simulink model "Vector_ComplexMult_Ex1"  (R2024a)
settings: Solver=VariableStepAuto  StartTime=0.0  StopTime=10  RelTol=1e-3
undefined symbols (not defined in the file): i, L, vsva2197, xcvc1702
libraries: hdlSSR x5, hdlBasic x4, vmcUtilities x1
settings Model: Creator=robg  LastModifiedBy=sdegala

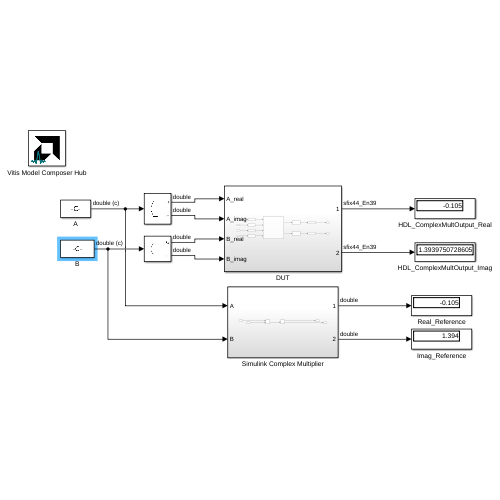
[thumbnail: Simulink's stored preview of the top-level diagram]
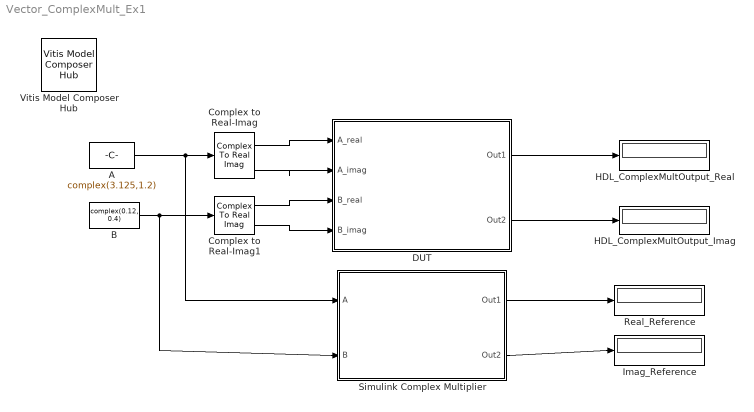
== system Vector_ComplexMult_Ex1 ==
  A : Constant  Value=complex(3.125,1.2)  SampleTime=1
  B : Constant  Value=complex(0.12, 0.4)  SampleTime=1
  Complex to Real-Imag : ComplexToRealImag
  Complex to Real-Imag1 : ComplexToRealImag
  DUT : Subsystem
  HDL_ComplexMultOutput_Imag : Display
  HDL_ComplexMultOutput_Real : Display
  Imag_Reference : Display
  Real_Reference : Display
  Simulink Complex Multiplier : Subsystem
  Vitis Model Composer Hub : vmcUtilities/Vitis Model Composer Hub  Tag=genX  CodeGeneration=off  CompilationType=HDLCompilation  ExportTypeV2=IP Catalog  StartColumn=1  NumberOfColumns=1  TargetDirectory=./netlist  exportDesign=off  analyzeDesign=off  validateDesignOnHw=off  ExportType=AI Engines  IpVendor=xilinx.com  IpLibrary=hls  IpVersion=1.0  IpHWLanguage=Verilog  AieCompilerOptions={}  AieSimulatorOptions={}  CreateTestbench=off  TestbenchStackSize=10  RunRtlSim=off  RunCSim=off  RunAieSim=off  AieSimTimeout=50000  RunAieSimProfiling=off  LaunchVitisAnalyzer=off  PlotOutput=off  RunX86Sim=off  X86SimTimeout=10  GenHwImage=off  GenLibadfXo=off  GenHwValidationCode=off  PlatformType=Not Specified  HwSystemType=Baremetal  HwValidationTarget=hw  ProjDevice=xcvc1702-vsva2197-1MP-i-L  ProjDevicePart=xcvc1702-vsva2197-1MP-i-L  AIEType=AIE  SamplePeriod=-1  ClockFrequency=200  DataPathParallelism=1  xilinxfamily=versalaicore  part=xcvc1702  speed=-1MP-i-L  package=vsva2197  directory=./netlist  testbench=off  incr_netlist=off  synthesis_tool=Vivado  clock_wrapper=Clock Enables  dbl_ovrd=According to Block Masks  dcm_input_clock_period=10  sysclk_period=10  simulink_period=1  eval_field=0  LogFileName=''  NThreads=4
  wires:
  Simulink Complex Multiplier/1(Out1) -> Real_Reference/1
  Simulink Complex Multiplier/2(Out2) -> Imag_Reference/1
  DUT/1(Out1) -> HDL_ComplexMultOutput_Real/1
  DUT/2(Out2) -> HDL_ComplexMultOutput_Imag/1
  A/1 -> Simulink Complex Multiplier/1(A), Complex to Real-Imag/1
  Complex to Real-Imag/1 -> DUT/1(A_real)
  Complex to Real-Imag/2 -> DUT/2(A_imag)
  B/1 -> Simulink Complex Multiplier/2(B), Complex to Real-Imag1/1
  Complex to Real-Imag1/1 -> DUT/3(B_real)
  Complex to Real-Imag1/2 -> DUT/4(B_imag)

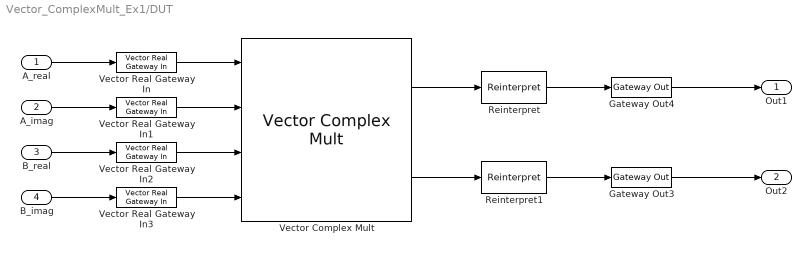
== system Vector_ComplexMult_Ex1/DUT ==
  A_real : Inport
  A_imag : Inport  Port=2
  B_real : Inport  Port=3
  B_imag : Inport  Port=4
  Gateway Out3 : hdlBasic/Gateway Out  inherit_from_input=on  bool_to_boolean=off  hdl_port=on  rows=1  columns=1  UseAsDAC=off  DACChannel='1'  interface=None  automatic_assignment=on  address_offset=hex2dec('00')  intf_name=''  intf_description=''  timing_constraint=None  locs_specified=off  LOCs={}  io_standard={}  XmcBlockStatus=1  maskContainerNames=group4  block_type=gatewayout  block_config=sysgen:gateway_out_config  block_width_w=590  block_height_w=620  block_width=620  block_height=750
  Gateway Out4 : hdlBasic/Gateway Out  inherit_from_input=on  bool_to_boolean=off  hdl_port=on  rows=1  columns=1  UseAsDAC=off  DACChannel='1'  interface=None  automatic_assignment=on  address_offset=hex2dec('00')  intf_name=''  intf_description=''  timing_constraint=None  locs_specified=off  LOCs={}  io_standard={}  XmcBlockStatus=1  maskContainerNames=group4  block_type=gatewayout  block_config=sysgen:gateway_out_config  block_width_w=590  block_height_w=620  block_width=620  block_height=750
  Reinterpret : hdlBasic/Reinterpret  force_arith_type=off  arith_type=Unsigned  force_bin_pt=on  bin_pt=39  XmcBlockStatus=1  maskContainerNames=group1  block_type=reinterpret  block_config=sysgen:Reinterpret_config
  Reinterpret1 : hdlBasic/Reinterpret  force_arith_type=off  arith_type=Unsigned  force_bin_pt=on  bin_pt=39  XmcBlockStatus=1  maskContainerNames=group1  block_type=reinterpret  block_config=sysgen:Reinterpret_config
  Vector Complex Mult : hdlSSR/Vector Complex Mult  sg_ssr=1  use_synth_mdl=off  block_type=cmplxmult_ssr  XmcBlockStatus=1  sg_ssr_prev=1  maskContainerNames=group1
  Vector Real Gateway In : hdlSSR/Vector Real Gateway In  gui_display_data_type=Fixed-point  arith_type=Signed (2's comp)  n_bits=26  bin_pt=23  preci_type=Single  exp_width=8  frac_width=24  quantization="Round  (unbiased: +/- Inf)"  overflow=Saturate  period=1  sg_ssr=1  UseAsADC=off  ADCChannel='1'  interface=None  automatic_assignment=on  address_offset=hex2dec('00')  intf_name=''  intf_description=''  default_value=0  timing_constraint=None  locs_specified=off  LOCs={}  io_standard={}  inherit_from_input=off  hdl_port=on  interface_prev=1  block_type=realgatewayin_ssr  XmcBlockStatus=1  sg_ssr_prev=1  maskContainerNames=group4  block_width_w=590  block_height_w=670  block_width=640  block_height=850
  Vector Real Gateway In1 : hdlSSR/Vector Real Gateway In  gui_display_data_type=Fixed-point  arith_type=Signed (2's comp)  n_bits=26  bin_pt=23  preci_type=Single  exp_width=8  frac_width=24  quantization="Round  (unbiased: +/- Inf)"  overflow=Saturate  period=1  sg_ssr=1  UseAsADC=off  ADCChannel='1'  interface=None  automatic_assignment=on  address_offset=hex2dec('00')  intf_name=''  intf_description=''  default_value=0  timing_constraint=None  locs_specified=off  LOCs={}  io_standard={}  inherit_from_input=off  hdl_port=on  interface_prev=1  block_type=realgatewayin_ssr  XmcBlockStatus=1  sg_ssr_prev=1  maskContainerNames=group4  block_width_w=590  block_height_w=670  block_width=640  block_height=850
  Vector Real Gateway In2 : hdlSSR/Vector Real Gateway In  gui_display_data_type=Fixed-point  arith_type=Signed (2's comp)  n_bits=18  bin_pt=16  preci_type=Single  exp_width=8  frac_width=24  quantization="Round  (unbiased: +/- Inf)"  overflow=Saturate  period=1  sg_ssr=1  UseAsADC=off  ADCChannel='1'  interface=None  automatic_assignment=on  address_offset=hex2dec('00')  intf_name=''  intf_description=''  default_value=0  timing_constraint=None  locs_specified=off  LOCs={}  io_standard={}  inherit_from_input=off  hdl_port=on  interface_prev=1  block_type=realgatewayin_ssr  XmcBlockStatus=1  sg_ssr_prev=1  maskContainerNames=group4  block_width_w=590  block_height_w=670  block_width=640  block_height=850
  Vector Real Gateway In3 : hdlSSR/Vector Real Gateway In  gui_display_data_type=Fixed-point  arith_type=Signed (2's comp)  n_bits=18  bin_pt=16  preci_type=Single  exp_width=8  frac_width=24  quantization="Round  (unbiased: +/- Inf)"  overflow=Saturate  period=1  sg_ssr=1  UseAsADC=off  ADCChannel='1'  interface=None  automatic_assignment=on  address_offset=hex2dec('00')  intf_name=''  intf_description=''  default_value=0  timing_constraint=None  locs_specified=off  LOCs={}  io_standard={}  inherit_from_input=off  hdl_port=on  interface_prev=1  block_type=realgatewayin_ssr  XmcBlockStatus=1  sg_ssr_prev=1  maskContainerNames=group4  block_width_w=590  block_height_w=670  block_width=640  block_height=850
  Out1 : Outport
  Out2 : Outport  Port=2
  wires:
  Gateway Out3/1 -> Out2/1
  Gateway Out4/1 -> Out1/1
  Vector Complex Mult/2 -> Reinterpret1/1
  Reinterpret/1 -> Gateway Out4/1
  Vector Complex Mult/1 -> Reinterpret/1
  A_real/1 -> Vector Real Gateway In/1
  Vector Real Gateway In/1 -> Vector Complex Mult/1
  Reinterpret1/1 -> Gateway Out3/1
  B_real/1 -> Vector Real Gateway In2/1
  Vector Real Gateway In2/1 -> Vector Complex Mult/3
  A_imag/1 -> Vector Real Gateway In1/1
  Vector Real Gateway In1/1 -> Vector Complex Mult/2
  B_imag/1 -> Vector Real Gateway In3/1
  Vector Real Gateway In3/1 -> Vector Complex Mult/4

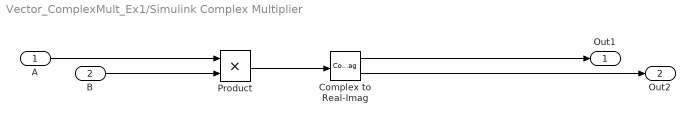
== system Vector_ComplexMult_Ex1/Simulink Complex Multiplier ==
  A : Inport
  B : Inport  Port=2
  Complex to Real-Imag : ComplexToRealImag
  Product : Product
  Out1 : Outport
  Out2 : Outport  Port=2
  wires:
  Product/1 -> Complex to Real-Imag/1
  Complex to Real-Imag/1 -> Out1/1
  Complex to Real-Imag/2 -> Out2/1
  A/1 -> Product/1
  B/1 -> Product/2
